simulink model "BLDCmotorControl_FOC_R2017b_fixdt_speedDeriv"  (R2025a)
settings: Solver=FixedStepDiscrete  StartTime=0  StopTime=0.5  FixedStep=Ts  MaxStep=1e-6  RelTol=1e-6  AbsTol=1e-6  EnableMultiTasking=on
PreLoadFcn:
  | addpath(genpath('01_Libraries'));
  | addpath(genpath('02_Figures'));
InitFcn:
  | init_model;
undefined symbols (not defined in the file): a_elecAngle, b_DCLinkCurrAvail, b_fieldWeakEna, b_selPhaABCurrMeas, cf_currFilt, cf_speedCoef, CTRL_COM, DiscIntNeverNeededParam, dV_openRate, DWORK0, DWORK1, DWORK2, DWORK3, dz_cntTrnsDetHi, dz_cntTrnsDetLo, i_max, i_qMax_M1, i_thresOutlier, id_fieldWeak_M1, id_Kb, id_Ki, id_Kp, iq_Kb, iq_Ki, iq_Kp, iq_KpLimProt, n_commAcvLo, n_commDeacvHi, n_Kb, n_Ki, n_Kp, n_KpLimProt, n_max, n_stdStillDet, OPEN_MODE, r_cos_M1, r_sin_M1, r_whl, SPD_MODE, TRQ_MODE, Ts, Ts_ctrl, V_dMax, V_max, V_min, V_qMax_M1, vec_hallToPos, VLT_MODE, z_commutMap_M1, z_ctrlModReq, z_ctrlTypSel, z_maxCntRst
libraries: simulink x11, BLDC_controller_Lib x9, spsVoltageMeasurementLib x2, simulink_extras x1, spsControlledVoltageSourceLib x1, spsPermanentMagnetSynchronousMachineLib x1, spsUniversalBridgeLib x1, spspowerguiLib x1, eePwmGenerator x1, SignalEditorBlockLib x1
(part 3 of 3)

== system BLDCmotorControl_FOC_R2017b_fixdt_speedDeriv/BLDC_controller/BLDC_controller/F03_Field_Oriented_Control/Open_Mode ==
  note: This will reduce the control command to 0 with a predefined rate.
  V_qPrev : Inport
  Action Port : ActionPort  InitializeStates=reset  ActionPortLabel=default: { }
  Constant23 : Constant  Value=0  OutDataTypeStr=Inherit: Inherit via back propagation
  Data Type Conversion : DataTypeConversion  OutDataTypeStr=fixdt(1,28,16)  SaturateOnIntegerOverflow=off  RndMeth=Floor
  Gain3 : Gain  Tag=struct('comment',struct('text','','placement',1),'logdata',struct('maxnumvals',inf,'plotchannels',[],'loggingmode',3,'channels',1),'output',struct('variable','','description','','name','$S_$B','width',1,'address','','max',NaN,'min',NaN,'class','default','type','CONTINUOUS','scaling','','lsb',1,'offset',0,'arb',0,'freeze',1,'unit','','autoscalingmode',1,'lowerheadroom',1,'upperheadroom',1,'headroomunit','bit','keepdatatype',1,'checkmin',0,'checkmax',0,'castoutput',0,'show',0),'gain',struct('variable','','description','','name','$S_$B_gain','width',1,'address','','max',NaN,'min',NaN,'class','default','type','CONTINUOUS','scaling','','lsb',1,'offset',0,'arb',0,'freeze',1,'unit','','keepdatatype',1,'value','1','scalar',0,'tolerance',1),'scalingvalid',0,'date',730486)  Gain=-1  RndMeth=Zero  OutDataTypeStr=Inherit: Same as input
  Rate_Limiter : BLDC_controller_Lib/Rate_Limiter  SystemSampleTime=-1  VariantActivationTime=update diagram  EmptyChoice=off  PassThrough=off  PassThroughVariantControl=(default)  EmptyChoiceVariantControl=(default)  AllowFlexibleInterface=on  Latency=0  AutoFrameSizeCalculation=off
  dV_openRate : Constant  Value=dV_openRate  OutDataTypeStr=fixdt(1,28,16)
  for merge : Gain  Tag=struct('comment',struct('text','','placement',1),'logdata',struct('maxnumvals',inf,'plotchannels',[],'loggingmode',3,'channels',1),'output',struct('variable','','description','','name','$S_$B','width',1,'address','','max',NaN,'min',NaN,'class','default','type','CONTINUOUS','scaling','','lsb',1,'offset',0,'arb',0,'freeze',1,'unit','','autoscalingmode',1,'lowerheadroom',1,'upperheadroom',1,'headroomunit','bit','keepdatatype',1,'checkmin',0,'checkmax',0,'castoutput',0,'show',0),'gain',struct('variable','','description','','name','$S_$B_gain','width',1,'address','','max',NaN,'min',NaN,'class','default','type','CONTINUOUS','scaling','','lsb',1,'offset',0,'arb',0,'freeze',1,'unit','','keepdatatype',1,'value','1','scalar',0,'tolerance',1),'scalingvalid',0,'date',730486)  OutDataTypeStr=fixdt(1,16,4)  RndMeth=Zero
  rising_edge_init : BLDC_controller_Lib/rising_edge_init
  V_qOpen : Outport  VectorParamsAs1DForOutWhenUnconnected=off
  wires:
  V_qPrev/1 -> [V_qPrev]
  Constant23/1 -> Rate_Limiter/1
  rising_edge_init/1 -> Rate_Limiter/3
  Gain3/1 -> Rate_Limiter/5
  dV_openRate/1 -> Gain3/1, Rate_Limiter/4
  for merge/1 -> [V_qOpen]
  [V_qOpen] -> V_qOpen/1
  Rate_Limiter/1 -> for merge/1
  [V_qPrev] -> Data Type Conversion/1
  Data Type Conversion/1 -> Rate_Limiter/2

== system BLDCmotorControl_FOC_R2017b_fixdt_speedDeriv/BLDC_controller/BLDC_controller/F03_Field_Oriented_Control/Outliers_Removal_and_Filtering ==
  i_qRaw : Inport
  i_dRaw : Inport  Port=2
  i_DCLink : Inport  Port=3
  DCLink_Current_Available : Subsystem
  DCLink_Current_NOT_Available : Subsystem
  If1 : If  IfExpression=u1 ~= 0
  Merge : Merge
  Merge1 : Merge
  b_DCLinkCurrAvail : Constant  Value=b_DCLinkCurrAvail  OutDataTypeStr=boolean
  i_q : Outport  VectorParamsAs1DForOutWhenUnconnected=off
  i_d : Outport  Port=2  VectorParamsAs1DForOutWhenUnconnected=off
  wires:
  [i_d] -> i_d/1
  [i_q] -> i_q/1
  i_qRaw/1 -> [i_qRaw]
  i_dRaw/1 -> [i_dRaw]
  [i_qRaw] -> DCLink_Current_NOT_Available/1(i_qRaw)
  [i_dRaw] -> DCLink_Current_NOT_Available/2(i_dRaw)
  If1/1 -> DCLink_Current_Available/Action
  i_DCLink/1 -> [i_DCLink]
  [i_dRaw] -> DCLink_Current_Available/2(i_dRaw)
  [i_qRaw] -> DCLink_Current_Available/1(i_qRaw)
  [i_DCLink] -> DCLink_Current_Available/3(i_DCLink)
  b_DCLinkCurrAvail/1 -> If1/1
  DCLink_Current_NOT_Available/1(i_qNoDCLink) -> [i_qNoDCLink]
  DCLink_Current_NOT_Available/2(i_dNoDCLink) -> [i_dNoDCLink]
  DCLink_Current_Available/1(i_qDCLink) -> [i_qDCLink]
  DCLink_Current_Available/2(i_dDCLink) -> [i_dDCLink]
  Merge1/1 -> [i_d]
  If1/2 -> DCLink_Current_NOT_Available/Action
  [i_qNoDCLink] -> Merge/2
  [i_qDCLink] -> Merge/1
  [i_dDCLink] -> Merge1/1
  [i_dNoDCLink] -> Merge1/2
  Merge/1 -> [i_q]

== system BLDCmotorControl_FOC_R2017b_fixdt_speedDeriv/BLDC_controller/BLDC_controller/F03_Field_Oriented_Control/Park_Transform ==
  note: Park Transform:
      | i_q = -i_alpha*sin(angle) + i_beta*cos(angle)
      | i_d = i_alpha*cos(angle) + i_beta*sin(angle)
  i_apha : Inport
  i_beta : Inport  Port=2
  r_sin : Inport  Port=3
  r_cos : Inport  Port=4
  Divide{1..4} (4 alike) : Product  Inputs=**  RndMeth=Simplest
  Sum1 : Sum  OutDataTypeStr=fixdt(1,16,4)  RndMeth=Simplest  SaturateOnIntegerOverflow=on
  Sum6 : Sum  Inputs=-+  OutDataTypeStr=fixdt(1,16,4)  RndMeth=Simplest  SaturateOnIntegerOverflow=on
  i_q : Outport  VectorParamsAs1DForOutWhenUnconnected=off
  i_d : Outport  Port=2  VectorParamsAs1DForOutWhenUnconnected=off
  wires:
  r_sin/1 -> [r_sin]
  i_beta/1 -> [i_beta]
  i_apha/1 -> [i_apha]
  r_cos/1 -> [r_cos]
  [r_sin] -> Divide4/2
  [i_apha] -> Divide4/1
  Divide4/1 -> Sum6/1
  Divide1/1 -> Sum6/2
  [i_beta] -> Divide1/1
  [r_cos] -> Divide1/2
  Sum6/1 -> i_q/1
  Divide2/1 -> Sum1/1
  [i_apha] -> Divide2/1
  [r_cos] -> Divide2/2
  Divide3/1 -> Sum1/2
  [i_beta] -> Divide3/1
  [r_sin] -> Divide3/2
  Sum1/1 -> i_d/1

== system BLDCmotorControl_FOC_R2017b_fixdt_speedDeriv/BLDC_controller/BLDC_controller/F03_Field_Oriented_Control/Preliminary_Calculations ==
  note: Sine/Cosine Look-up Tables
  note: Field Weakening map as a function of the Motor Speed
  note: FOC Field weakening
  note: Note: The Sine and Cosine maps are shifted in phase by 30 deg to align with the Hall sensors position.
  a_elecAngle : Inport
  n_motAbs : Inport  Port=2
  Data Type Conversion : DataTypeConversion  OutDataTypeStr=fixdt(1,16,4)  SaturateOnIntegerOverflow=off  RndMeth=Floor
  Switch_PhaAdv1 : Switch  Criteria=u2 ~= 0  OutDataTypeStr=Inherit: Inherit via back propagation  RndMeth=Zero  SaturateOnIntegerOverflow=off  InputSameDT=off
  a_elecAngle_XA : PreLookup  BreakpointsData=a_elecAngle_XA  IndexSearchMethod=Evenly spaced points  BeginIndexSearchUsingPreviousIndexResult=on  IndexDataTypeStr=uint8  FractionDataTypeStr=fixdt(0,16,14)  RndMeth=Simplest
  a_elecPeriod2 : Constant  Value=0  OutDataTypeStr=Inherit: Inherit via back propagation
  b_fieldWeakEna : Constant  Value=b_fieldWeakEna  OutDataTypeStr=boolean
  id_fieldWeak_M1 : Interpolation_n-D  NumberOfTableDimensions=1  Table=id_fieldWeak_M1  ExtrapMethod=Clip  OutDataTypeStr=fixdt(0,10,0)  InternalRulePriority=Speed  RndMeth=Simplest
      settings: InputPortMap=u0,u1
  n_fieldWeak_XA : PreLookup  BreakpointsData=n_fieldWeak_XA  IndexSearchMethod=Evenly spaced points  BeginIndexSearchUsingPreviousIndexResult=on  IndexDataTypeStr=uint8  FractionDataTypeStr=fixdt(0,16,14)  RndMeth=Simplest
  r_cos_M1 : Interpolation_n-D  NumberOfTableDimensions=1  Table=r_cos_M1  ExtrapMethod=Clip  OutDataTypeStr=fixdt(1,16,14)  InternalRulePriority=Speed  RndMeth=Simplest
      settings: InputPortMap=u0,u1
  r_sin_M1 : Interpolation_n-D  NumberOfTableDimensions=1  Table=r_sin_M1  ExtrapMethod=Clip  OutDataTypeStr=fixdt(1,16,14)  InternalRulePriority=Speed  RndMeth=Simplest
      settings: InputPortMap=u0,u1
  r_sin : Outport  VectorParamsAs1DForOutWhenUnconnected=off
  r_cos : Outport  Port=2  VectorParamsAs1DForOutWhenUnconnected=off
  i_dTgt : Outport  Port=3  VectorParamsAs1DForOutWhenUnconnected=off
  wires:
  a_elecAngle_XA/2 -> r_sin_M1/2, r_cos_M1/2
  a_elecAngle_XA/1 -> r_cos_M1/1, r_sin_M1/1
  r_sin_M1/1 -> r_sin/1
  a_elecAngle/1 -> a_elecAngle_XA/1
  r_cos_M1/1 -> r_cos/1
  n_fieldWeak_XA/1 -> id_fieldWeak_M1/1
  n_fieldWeak_XA/2 -> id_fieldWeak_M1/2
  id_fieldWeak_M1/1 -> Data Type Conversion/1
  n_motAbs/1 -> n_fieldWeak_XA/1
  b_fieldWeakEna/1 -> Switch_PhaAdv1/2
  a_elecPeriod2/1 -> Switch_PhaAdv1/3
  Switch_PhaAdv1/1 -> i_dTgt/1
  Data Type Conversion/1 -> Switch_PhaAdv1/1

== system BLDCmotorControl_FOC_R2017b_fixdt_speedDeriv/BLDC_controller/BLDC_controller/F03_Field_Oriented_Control/Speed_Mode ==
  r_DC : Inport
  V_qMax : Inport  Port=2
  V_qMin : Inport  Port=3
  n_mot : Inport  Port=4
  n_max : Inport  Port=5
  n_min : Inport  Port=6
  i_qLimProt : Inport  Port=7
  Action Port : ActionPort  InitializeStates=reset  ActionPortLabel=case: { }
  Gain5 : Gain  Tag=struct('comment',struct('text','','placement',1),'logdata',struct('maxnumvals',inf,'plotchannels',[],'loggingmode',3,'channels',1),'output',struct('variable','','description','','name','$S_$B','width',1,'address','','max',NaN,'min',NaN,'class','default','type','CONTINUOUS','scaling','','lsb',1,'offset',0,'arb',0,'freeze',1,'unit','','autoscalingmode',1,'lowerheadroom',1,'upperheadroom',1,'headroomunit','bit','keepdatatype',1,'checkmin',0,'checkmax',0,'castoutput',0,'show',0),'gain',struct('variable','','description','','name','$S_$B_gain','width',1,'address','','max',NaN,'min',NaN,'class','default','type','CONTINUOUS','scaling','','lsb',1,'offset',0,'arb',0,'freeze',1,'unit','','keepdatatype',1,'value','1','scalar',0,'tolerance',1),'scalingvalid',0,'date',730486)  Gain=-1  OutDataTypeStr=fixdt(1,16,4)  RndMeth=Zero  ParamDataTypeStr=Inherit: Same as input
  PI_backCalc_fixdt_n : BLDC_controller_Lib/PI_backCalc_fixdt  SystemSampleTime=-1  VariantActivationTime=update diagram  EmptyChoice=off  PassThrough=off  PassThroughVariantControl=(default)  EmptyChoiceVariantControl=(default)  AllowFlexibleInterface=on  Latency=0  AutoFrameSizeCalculation=off
  Saturation Dynamic1 : simulink/Discontinuities/Saturation Dynamic  OutMin=[]  OutMax=[]  OutDataTypeStr=Inherit: Same as second input  OutDataType=fixdt(1, 16)  OutScaling=2^-10  DoSatur=off
  Sum1 : Sum  RndMeth=Simplest
  Sum3 : Sum  Inputs=|+-  RndMeth=Simplest
  a_elecPeriod11 : Constant  Value=n_Kb  OutDataTypeStr=fixdt(0,16,16)
  a_elecPeriod15 : Constant  Value=n_Kp  OutDataTypeStr=fixdt(0,16,8)
  a_elecPeriod20 : Constant  Value=n_Ki  VectorParams1D=off  OutDataTypeStr=fixdt(0,16,16)
  V_qSpd : Outport  VectorParamsAs1DForOutWhenUnconnected=off
  wires:
  [V_qMin] -> PI_backCalc_fixdt_n/6
  [V_qMax] -> PI_backCalc_fixdt_n/5
  a_elecPeriod20/1 -> PI_backCalc_fixdt_n/3
  a_elecPeriod11/1 -> PI_backCalc_fixdt_n/4
  a_elecPeriod15/1 -> PI_backCalc_fixdt_n/2
  [n_mot] -> Sum3/2
  Sum3/1 -> PI_backCalc_fixdt_n/1
  r_DC/1 -> [r_DC]
  V_qMax/1 -> [V_qMax]
  V_qMin/1 -> [V_qMin]
  n_mot/1 -> [n_mot]
  PI_backCalc_fixdt_n/1 -> Sum1/1
  [V_qSpd] -> V_qSpd/1
  Gain5/1 -> [V_qSpd]
  [n_min] -> Saturation Dynamic1/3
  [n_max] -> Saturation Dynamic1/1
  [r_DC] -> Saturation Dynamic1/2
  Saturation Dynamic1/1 -> Sum3/1
  n_min/1 -> [n_min]
  n_max/1 -> [n_max]
  Sum1/1 -> Gain5/1
  i_qLimProt/1 -> [i_qLimProt]
  [i_qLimProt] -> Sum1/2

== system BLDCmotorControl_FOC_R2017b_fixdt_speedDeriv/BLDC_controller/BLDC_controller/F03_Field_Oriented_Control/Torque_Mode ==
  r_DC : Inport
  V_qMax : Inport  Port=2
  V_qMin : Inport  Port=3
  i_q : Inport  Port=4
  i_qMax : Inport  Port=5
  i_qMin : Inport  Port=6
  n_limProt : Inport  Port=7
  Action Port : ActionPort  InitializeStates=reset  ActionPortLabel=case: { }
  PI_backCalc_fixdt_Iq : BLDC_controller_Lib/PI_backCalc_fixdt  SystemSampleTime=-1  VariantActivationTime=update diagram  EmptyChoice=off  PassThrough=off  PassThroughVariantControl=(default)  EmptyChoiceVariantControl=(default)  AllowFlexibleInterface=on  Latency=0  AutoFrameSizeCalculation=off
  Saturation Dynamic : simulink/Discontinuities/Saturation Dynamic  OutMin=[]  OutMax=[]  OutDataTypeStr=Inherit: Same as second input  OutDataType=fixdt(1, 16)  OutScaling=2^-10  DoSatur=off
  Sum1 : Sum  Inputs=|+-  RndMeth=Simplest
  Sum2 : Sum  RndMeth=Simplest
  a_elecPeriod10 : Constant  Value=iq_Kb  OutDataTypeStr=fixdt(0,16,16)
  a_elecPeriod12 : Constant  Value=iq_Kp  OutDataTypeStr=fixdt(0,16,8)
  a_elecPeriod13 : Constant  Value=iq_Ki  OutDataTypeStr=fixdt(0,16,16)
  due_to_conv : Gain  Tag=struct('comment',struct('text','','placement',1),'logdata',struct('maxnumvals',inf,'plotchannels',[],'loggingmode',3,'channels',1),'output',struct('variable','','description','','name','$S_$B','width',1,'address','','max',NaN,'min',NaN,'class','default','type','CONTINUOUS','scaling','','lsb',1,'offset',0,'arb',0,'freeze',1,'unit','','autoscalingmode',1,'lowerheadroom',1,'upperheadroom',1,'headroomunit','bit','keepdatatype',1,'checkmin',0,'checkmax',0,'castoutput',0,'show',0),'gain',struct('variable','','description','','name','$S_$B_gain','width',1,'address','','max',NaN,'min',NaN,'class','default','type','CONTINUOUS','scaling','','lsb',1,'offset',0,'arb',0,'freeze',1,'unit','','keepdatatype',1,'value','1','scalar',0,'tolerance',1),'scalingvalid',0,'date',730486)  Gain=-1  OutDataTypeStr=fixdt(1,16,3)  RndMeth=Zero  ParamDataTypeStr=Inherit: Same as input
  for merge : Gain  Tag=struct('comment',struct('text','','placement',1),'logdata',struct('maxnumvals',inf,'plotchannels',[],'loggingmode',3,'channels',1),'output',struct('variable','','description','','name','$S_$B','width',1,'address','','max',NaN,'min',NaN,'class','default','type','CONTINUOUS','scaling','','lsb',1,'offset',0,'arb',0,'freeze',1,'unit','','autoscalingmode',1,'lowerheadroom',1,'upperheadroom',1,'headroomunit','bit','keepdatatype',1,'checkmin',0,'checkmax',0,'castoutput',0,'show',0),'gain',struct('variable','','description','','name','$S_$B_gain','width',1,'address','','max',NaN,'min',NaN,'class','default','type','CONTINUOUS','scaling','','lsb',1,'offset',0,'arb',0,'freeze',1,'unit','','keepdatatype',1,'value','1','scalar',0,'tolerance',1),'scalingvalid',0,'date',730486)  RndMeth=Zero  OutDataTypeStr=Inherit: Same as input  ParamDataTypeStr=Inherit: Same as input
  V_qTrq : Outport  VectorParamsAs1DForOutWhenUnconnected=off
  wires:
  a_elecPeriod13/1 -> PI_backCalc_fixdt_Iq/3
  [r_DC] -> Sum2/1
  Saturation Dynamic/1 -> Sum1/1
  [V_qMax] -> PI_backCalc_fixdt_Iq/5
  [V_qMin] -> PI_backCalc_fixdt_Iq/6
  [i_q] -> Sum1/2
  Sum1/1 -> PI_backCalc_fixdt_Iq/1
  a_elecPeriod10/1 -> PI_backCalc_fixdt_Iq/4
  a_elecPeriod12/1 -> PI_backCalc_fixdt_Iq/2
  V_qMax/1 -> [V_qMax]
  r_DC/1 -> [r_DC]
  V_qMin/1 -> [V_qMin]
  i_q/1 -> [i_q]
  [V_qTrq] -> V_qTrq/1
  PI_backCalc_fixdt_Iq/1 -> for merge/1
  for merge/1 -> [V_qTrq]
  i_qMin/1 -> [i_qMin]
  i_qMax/1 -> [i_qMax]
  [i_qMin] -> Saturation Dynamic/3
  [i_qMax] -> Saturation Dynamic/1
  due_to_conv/1 -> Saturation Dynamic/2
  [n_limProt] -> Sum2/2
  n_limProt/1 -> [n_limProt]
  Sum2/1 -> due_to_conv/1

== system BLDCmotorControl_FOC_R2017b_fixdt_speedDeriv/BLDC_controller/BLDC_controller/F03_Field_Oriented_Control/Vd_Calculation ==
  i_dTgt : Inport
  i_d : Inport  Port=2
  V_dMax : Inport  Port=3
  V_dMin : Inport  Port=4
  i_dMax : Inport  Port=5
  i_dMin : Inport  Port=6
  Action Port : ActionPort  InitializeStates=reset  ActionPortLabel=if { }
  PI_backCalc_fixdt_Id : BLDC_controller_Lib/PI_backCalc_fixdt  SystemSampleTime=-1  VariantActivationTime=update diagram  EmptyChoice=off  PassThrough=off  PassThroughVariantControl=(default)  EmptyChoiceVariantControl=(default)  AllowFlexibleInterface=on  Latency=0  AutoFrameSizeCalculation=off
  Saturation Dynamic : simulink/Discontinuities/Saturation Dynamic  OutMin=[]  OutMax=[]  OutDataTypeStr=Inherit: Same as second input  OutDataType=fixdt(1, 16)  OutScaling=2^-10  DoSatur=off
  Sum3 : Sum  Inputs=|+-  RndMeth=Simplest
  a_elecPeriod11 : Constant  Value=id_Kb  OutDataTypeStr=fixdt(0,16,16)
  a_elecPeriod6 : Constant  Value=id_Kp  OutDataTypeStr=fixdt(0,16,8)
  a_elecPeriod7 : Constant  Value=id_Ki  OutDataTypeStr=fixdt(0,16,16)
  V_d : Outport  OutputWhenDisabled=reset  InitialOutput=0  VectorParamsAs1DForOutWhenUnconnected=off
  wires:
  a_elecPeriod6/1 -> PI_backCalc_fixdt_Id/2
  Sum3/1 -> PI_backCalc_fixdt_Id/1
  [V_dMin] -> PI_backCalc_fixdt_Id/6
  [V_dMax] -> PI_backCalc_fixdt_Id/5
  a_elecPeriod7/1 -> PI_backCalc_fixdt_Id/3
  a_elecPeriod11/1 -> PI_backCalc_fixdt_Id/4
  PI_backCalc_fixdt_Id/1 -> [V_d]
  [i_d] -> Sum3/2
  [i_dTgt] -> Saturation Dynamic/2
  [V_d] -> V_d/1
  i_dTgt/1 -> [i_dTgt]
  i_d/1 -> [i_d]
  V_dMin/1 -> [V_dMin]
  V_dMax/1 -> [V_dMax]
  i_dMax/1 -> [i_dMax]
  i_dMin/1 -> [i_dMin]
  Saturation Dynamic/1 -> Sum3/1
  [i_dMax] -> Saturation Dynamic/1
  [i_dMin] -> Saturation Dynamic/3

== system BLDCmotorControl_FOC_R2017b_fixdt_speedDeriv/BLDC_controller/BLDC_controller/F03_Field_Oriented_Control/Voltage_Mode ==
  r_DC : Inport
  V_qMax : Inport  Port=2
  V_qMin : Inport  Port=3
  i_qLimProt : Inport  Port=4
  n_limProt : Inport  Port=5
  Action Port : ActionPort  InitializeStates=reset  ActionPortLabel=case: { }
  Saturation Dynamic1 : simulink/Discontinuities/Saturation Dynamic  OutMin=[]  OutMax=[]  OutDataTypeStr=Inherit: Same as second input  OutDataType=fixdt(1, 16)  OutScaling=2^-10  DoSatur=off
  Sum3 : Sum  Inputs=+++  RndMeth=Simplest
  due_to_conv : Gain  Tag=struct('comment',struct('text','','placement',1),'logdata',struct('maxnumvals',inf,'plotchannels',[],'loggingmode',3,'channels',1),'output',struct('variable','','description','','name','$S_$B','width',1,'address','','max',NaN,'min',NaN,'class','default','type','CONTINUOUS','scaling','','lsb',1,'offset',0,'arb',0,'freeze',1,'unit','','autoscalingmode',1,'lowerheadroom',1,'upperheadroom',1,'headroomunit','bit','keepdatatype',1,'checkmin',0,'checkmax',0,'castoutput',0,'show',0),'gain',struct('variable','','description','','name','$S_$B_gain','width',1,'address','','max',NaN,'min',NaN,'class','default','type','CONTINUOUS','scaling','','lsb',1,'offset',0,'arb',0,'freeze',1,'unit','','keepdatatype',1,'value','1','scalar',0,'tolerance',1),'scalingvalid',0,'date',730486)  Gain=-1  OutDataTypeStr=fixdt(1,16,4)  RndMeth=Zero  ParamDataTypeStr=Inherit: Same as input
  V_qVlt : Outport  VectorParamsAs1DForOutWhenUnconnected=off
  wires:
  r_DC/1 -> [r_DC]
  [V_qMin] -> Saturation Dynamic1/3
  [V_qMax] -> Saturation Dynamic1/1
  [V_qVlt] -> V_qVlt/1
  V_qMax/1 -> [V_qMax]
  V_qMin/1 -> [V_qMin]
  Saturation Dynamic1/1 -> due_to_conv/1
  i_qLimProt/1 -> [i_qLimProt]
  [i_qLimProt] -> Sum3/2
  n_limProt/1 -> [n_limProt]
  [n_limProt] -> Sum3/3
  Sum3/1 -> Saturation Dynamic1/2
  due_to_conv/1 -> [V_qVlt]
  [r_DC] -> Sum3/1

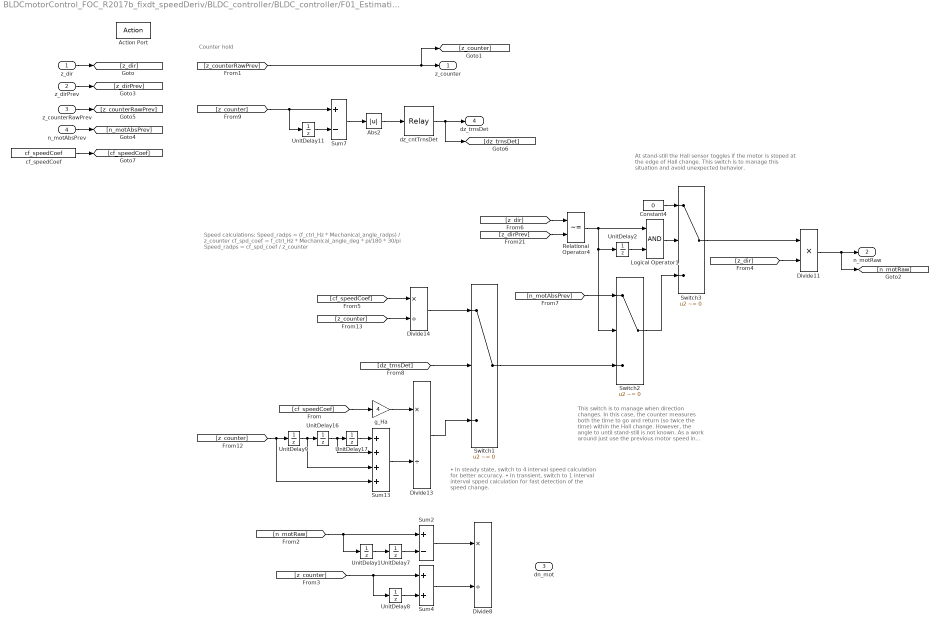
== system BLDCmotorControl_FOC_R2017b_fixdt_speedDeriv/BLDC_controller/BLDC_controller/F01_Estimations/F01_04_Speed_Estimation/Raw_Motor_Speed_Estimation ==
  note: Speed calculations:
      | Speed_radps = (f_ctrl_Hz * Mechanical_angle_radps) / z_counter
      | cf_spd_coef = f_ctrl_Hz * Mechanical_angle_deg * pi/180 * 30/pi
      | Speed_radps = cf_spd_coef / z_counter
  note: Counter hold
  note: • In steady state, switch to 4 interval speed calculation for better accuracy.
      | • In transient, switch to 1 interval interval spped calculation for fast detection of the speed change.
  note: This switch is to manage when direction changes. In this case, the counter measures both the time to go and return (so twice the time) within the Hall change. However, the angle to until stand-still is not known. As a work around just use the previous motor speed in absolute value.
  note: At stand-still the Hall sensor toggles if the motor is stoped at the edge of Hall change. This switch is to manage this situation and avoid unexpected behavior.
  z_dir : Inport
  z_dirPrev : Inport  Port=2
  z_counterRawPrev : Inport  Port=3
  n_motAbsPrev : Inport  Port=4
  Action Port : ActionPort  ActionPortLabel=if(u1 ~= 0)
  Abs2 : Abs  OutDataTypeStr=Inherit: Inherit via back propagation  RndMeth=Zero  SaturateOnIntegerOverflow=off
  Constant4 : Constant  Value=0  OutDataTypeStr=Inherit: Inherit via back propagation
  Divide11 : Product  Inputs=**  RndMeth=Simplest  OutDataTypeStr=Inherit: Same as first input
  Divide13 : Product  Inputs=*/  OutDataTypeStr=fixdt(1,16,4)  RndMeth=Simplest
  Divide14 : Product  Inputs=*/  OutDataTypeStr=fixdt(1,16,4)  RndMeth=Simplest
  Divide8 : Product  Inputs=*/  OutDataTypeStr=fixdt(1,16,6)  RndMeth=Simplest  SaturateOnIntegerOverflow=on
  Logical Operator1 : Logic  AllPortsSameDT=off  OutDataTypeStr=boolean
  Relational Operator4 : RelationalOperator  Operator=~=  OutDataTypeStr=boolean  RndMeth=Simplest  InputSameDT=off
  Sum13 : Sum  Inputs=++++  InputSameDT=on  RndMeth=Simplest  OutDataTypeStr=Inherit: Same as first input
  Sum2 : Sum  Inputs=+-  RndMeth=Simplest  OutDataTypeStr=Inherit: Same as first input
  Sum4 : Sum  RndMeth=Simplest  OutDataTypeStr=Inherit: Same as first input
  Sum7 : Sum  Inputs=+-  InputSameDT=on  RndMeth=Simplest  OutDataTypeStr=Inherit: Same as first input
  Switch1 : Switch  Tag=struct('comment',struct('text','','placement',1),'logdata',struct('maxnumvals',inf,'plotchannels',[],'loggingmode',3,'channels',1),'output',struct('variable','','description','','name','$S_$B','width',1,'address','','max',NaN,'min',NaN,'class','default','type','CONTINUOUS','scaling','','lsb',1,'offset',0,'arb',0,'freeze',1,'unit','','autoscalingmode',1,'lowerheadroom',1,'upperheadroom',1,'headroomunit','bit','keepdatatype',1,'checkmin',0,'checkmax',0,'castoutput',0,'show',0),'threshold',struct('variable','','description','','name','$S_$B_threshold','width',1,'address','','max',NaN,'min',NaN,'class','default','type','CONTINUOUS','scaling','','lsb',1,'offset',0,'arb',0,'freeze',1,'unit','','keepdatatype',1,'value','0','scalar',0,'criteria',3),'scalingvalid',0,'date',733087.49614628474,'inheritscaling',0)  Criteria=u2 ~= 0
      settings: AttributesFormatString=threshold=%<threshold>\nCriteria : %<Criteria>
  Switch2 : Switch  Tag=struct('comment',struct('text','','placement',1),'logdata',struct('maxnumvals',inf,'plotchannels',[],'loggingmode',3,'channels',1),'output',struct('variable','','description','','name','$S_$B','width',1,'address','','max',NaN,'min',NaN,'class','default','type','CONTINUOUS','scaling','','lsb',1,'offset',0,'arb',0,'freeze',1,'unit','','autoscalingmode',1,'lowerheadroom',1,'upperheadroom',1,'headroomunit','bit','keepdatatype',1,'checkmin',0,'checkmax',0,'castoutput',0,'show',0),'threshold',struct('variable','','description','','name','$S_$B_threshold','width',1,'address','','max',NaN,'min',NaN,'class','default','type','CONTINUOUS','scaling','','lsb',1,'offset',0,'arb',0,'freeze',1,'unit','','keepdatatype',1,'value','0','scalar',0,'criteria',3),'scalingvalid',0,'date',733087.49614628474,'inheritscaling',0)  Criteria=u2 ~= 0
      settings: AttributesFormatString=threshold=%<threshold>\nCriteria : %<Criteria>
  Switch3 : Switch  Tag=struct('comment',struct('text','','placement',1),'logdata',struct('maxnumvals',inf,'plotchannels',[],'loggingmode',3,'channels',1),'output',struct('variable','','description','','name','$S_$B','width',1,'address','','max',NaN,'min',NaN,'class','default','type','CONTINUOUS','scaling','','lsb',1,'offset',0,'arb',0,'freeze',1,'unit','','autoscalingmode',1,'lowerheadroom',1,'upperheadroom',1,'headroomunit','bit','keepdatatype',1,'checkmin',0,'checkmax',0,'castoutput',0,'show',0),'threshold',struct('variable','','description','','name','$S_$B_threshold','width',1,'address','','max',NaN,'min',NaN,'class','default','type','CONTINUOUS','scaling','','lsb',1,'offset',0,'arb',0,'freeze',1,'unit','','keepdatatype',1,'value','0','scalar',0,'criteria',3),'scalingvalid',0,'date',733087.49614628474,'inheritscaling',0)  Criteria=u2 ~= 0
      settings: AttributesFormatString=threshold=%<threshold>\nCriteria : %<Criteria>
  UnitDelay{1..2,7..9,11,16..17} (8 alike) : UnitDelay  SampleTime=-1  HasFrameUpgradeWarning=on
  cf_speedCoef : Constant  Value=cf_speedCoef  OutDataTypeStr=fixdt(0,16,0)
  dz_cntTrnsDet : Relay  OnSwitchValue=dz_cntTrnsDetHi  OffSwitchValue=dz_cntTrnsDetLo  OutDataTypeStr=boolean
  g_Ha : Gain  Gain=4  OutDataTypeStr=Inherit: Inherit via back propagation  RndMeth=Zero  ParamDataTypeStr=Inherit: Same as input
  z_counter : Outport  InitialOutput=z_maxCntRst  VectorParamsAs1DForOutWhenUnconnected=off
  n_motRaw : Outport  Port=2  VectorParamsAs1DForOutWhenUnconnected=off
  dn_mot : Outport  Port=3  VectorParamsAs1DForOutWhenUnconnected=off
  dz_trnsDet : Outport  Port=4  VectorParamsAs1DForOutWhenUnconnected=off
  wires:
  z_dir/1 -> [z_dir]
  z_dirPrev/1 -> [z_dirPrev]
  z_counterRawPrev/1 -> [z_counterRawPrev]
  UnitDelay1/1 -> UnitDelay7/1
  Divide11/1 -> [n_motRaw], n_motRaw/1
  Sum2/1 -> Divide8/1
  [z_counter] -> UnitDelay8/1, Sum4/1
  [n_motRaw] -> Sum2/1, UnitDelay1/1
  UnitDelay7/1 -> Sum2/2
  UnitDelay8/1 -> Sum4/2
  Sum4/1 -> Divide8/2
  [z_dir] -> Divide11/2
  UnitDelay16/1 -> Sum13/2, UnitDelay17/1
  UnitDelay9/1 -> Sum13/3, UnitDelay16/1
  [z_counter] -> Sum13/4, UnitDelay9/1
  [cf_speedCoef] -> g_Ha/1
  Sum13/1 -> Divide13/2
  g_Ha/1 -> Divide13/1
  [z_counter] -> Divide14/2
  [cf_speedCoef] -> Divide14/1
  UnitDelay11/1 -> Sum7/2
  [z_counter] -> Sum7/1, UnitDelay11/1
  Sum7/1 -> Abs2/1
  Abs2/1 -> dz_cntTrnsDet/1
  [dz_trnsDet] -> Switch1/2
  cf_speedCoef/1 -> [cf_speedCoef]
  UnitDelay17/1 -> Sum13/1
  [z_dir] -> Relational Operator4/1
  [z_dirPrev] -> Relational Operator4/2
  UnitDelay2/1 -> Logical Operator1/2
  Relational Operator4/1 -> Switch2/2, UnitDelay2/1, Logical Operator1/1
  Logical Operator1/1 -> Switch3/2
  Switch2/1 -> Switch3/3
  Constant4/1 -> Switch3/1
  Switch3/1 -> Divide11/1
  Switch1/1 -> Switch2/3
  n_motAbsPrev/1 -> [n_motAbsPrev]
  [n_motAbsPrev] -> Switch2/1
  [z_counterRawPrev] -> [z_counter], z_counter/1
  dz_cntTrnsDet/1 -> [dz_trnsDet], dz_trnsDet/1
  Divide14/1 -> Switch1/1
  Divide13/1 -> Switch1/3

== system BLDCmotorControl_FOC_R2017b_fixdt_speedDeriv/BLDC_controller/BLDC_controller/F03_Field_Oriented_Control/Clarke_Transform/Clarke_PhasesAB ==
  note: Clarke Transform:
      | i_alpha = i_phaA
      | i_beta = ((1/sqrt(3))*i_phaA + (2/sqrt(3))*i_phaB)
  i_phaA : Inport
  i_phaB : Inport  Port=2
  Action Port : ActionPort  ActionPortLabel=if(u1 ~= 0)
  Gain2 : Gain  Tag=struct('comment',struct('text','','placement',1),'logdata',struct('maxnumvals',inf,'plotchannels',[],'loggingmode',3,'channels',1),'output',struct('variable','','description','','name','$S_$B','width',1,'address','','max',NaN,'min',NaN,'class','default','type','CONTINUOUS','scaling','','lsb',1,'offset',0,'arb',0,'freeze',1,'unit','','autoscalingmode',1,'lowerheadroom',1,'upperheadroom',1,'headroomunit','bit','keepdatatype',1,'checkmin',0,'checkmax',0,'castoutput',0,'show',0),'gain',struct('variable','','description','','name','$S_$B_gain','width',1,'address','','max',NaN,'min',NaN,'class','default','type','CONTINUOUS','scaling','','lsb',1,'offset',0,'arb',0,'freeze',1,'unit','','keepdatatype',1,'value','1','scalar',0,'tolerance',1),'scalingvalid',0,'date',730486)  Gain=2/sqrt(3)  RndMeth=Zero
  Gain4 : Gain  Tag=struct('comment',struct('text','','placement',1),'logdata',struct('maxnumvals',inf,'plotchannels',[],'loggingmode',3,'channels',1),'output',struct('variable','','description','','name','$S_$B','width',1,'address','','max',NaN,'min',NaN,'class','default','type','CONTINUOUS','scaling','','lsb',1,'offset',0,'arb',0,'freeze',1,'unit','','autoscalingmode',1,'lowerheadroom',1,'upperheadroom',1,'headroomunit','bit','keepdatatype',1,'checkmin',0,'checkmax',0,'castoutput',0,'show',0),'gain',struct('variable','','description','','name','$S_$B_gain','width',1,'address','','max',NaN,'min',NaN,'class','default','type','CONTINUOUS','scaling','','lsb',1,'offset',0,'arb',0,'freeze',1,'unit','','keepdatatype',1,'value','1','scalar',0,'tolerance',1),'scalingvalid',0,'date',730486)  Gain=1/sqrt(3)  RndMeth=Zero
  Sum1 : Sum  OutDataTypeStr=fixdt(1,16,4)  RndMeth=Simplest  SaturateOnIntegerOverflow=on
  for merge : Gain  Tag=struct('comment',struct('text','','placement',1),'logdata',struct('maxnumvals',inf,'plotchannels',[],'loggingmode',3,'channels',1),'output',struct('variable','','description','','name','$S_$B','width',1,'address','','max',NaN,'min',NaN,'class','default','type','CONTINUOUS','scaling','','lsb',1,'offset',0,'arb',0,'freeze',1,'unit','','autoscalingmode',1,'lowerheadroom',1,'upperheadroom',1,'headroomunit','bit','keepdatatype',1,'checkmin',0,'checkmax',0,'castoutput',0,'show',0),'gain',struct('variable','','description','','name','$S_$B_gain','width',1,'address','','max',NaN,'min',NaN,'class','default','type','CONTINUOUS','scaling','','lsb',1,'offset',0,'arb',0,'freeze',1,'unit','','keepdatatype',1,'value','1','scalar',0,'tolerance',1),'scalingvalid',0,'date',730486)  RndMeth=Zero  OutDataTypeStr=Inherit: Same as input  ParamDataTypeStr=Inherit: Same as input
  i_alphaAB : Outport  VectorParamsAs1DForOutWhenUnconnected=off
  i_betaAB : Outport  Port=2  VectorParamsAs1DForOutWhenUnconnected=off
  wires:
  i_phaB/1 -> [i_phaB]
  i_phaA/1 -> [i_phaA]
  [i_phaA] -> for merge/1, Gain4/1
  Gain2/1 -> Sum1/2
  [i_phaB] -> Gain2/1
  Gain4/1 -> Sum1/1
  Sum1/1 -> i_betaAB/1
  for merge/1 -> i_alphaAB/1

== system BLDCmotorControl_FOC_R2017b_fixdt_speedDeriv/BLDC_controller/BLDC_controller/F03_Field_Oriented_Control/Clarke_Transform/Clarke_PhasesBC ==
  note: Clarke Transform:
      | i_alpha = - i_phaB - i_phaC
      | i_beta = (1/sqrt(3)) * (i_phaB - i_phaC)
  i_phaB : Inport
  i_phaC : Inport  Port=2
  Action Port : ActionPort  ActionPortLabel=else
  Gain2 : Gain  Tag=struct('comment',struct('text','','placement',1),'logdata',struct('maxnumvals',inf,'plotchannels',[],'loggingmode',3,'channels',1),'output',struct('variable','','description','','name','$S_$B','width',1,'address','','max',NaN,'min',NaN,'class','default','type','CONTINUOUS','scaling','','lsb',1,'offset',0,'arb',0,'freeze',1,'unit','','autoscalingmode',1,'lowerheadroom',1,'upperheadroom',1,'headroomunit','bit','keepdatatype',1,'checkmin',0,'checkmax',0,'castoutput',0,'show',0),'gain',struct('variable','','description','','name','$S_$B_gain','width',1,'address','','max',NaN,'min',NaN,'class','default','type','CONTINUOUS','scaling','','lsb',1,'offset',0,'arb',0,'freeze',1,'unit','','keepdatatype',1,'value','1','scalar',0,'tolerance',1),'scalingvalid',0,'date',730486)  Gain=1/sqrt(3)  OutDataTypeStr=fixdt(1,16,4)  RndMeth=Zero  SaturateOnIntegerOverflow=on
  Sum1 : Sum  Inputs=--  OutDataTypeStr=fixdt(1,16,4)  RndMeth=Simplest  SaturateOnIntegerOverflow=on
  Sum3 : Sum  Inputs=+-  RndMeth=Simplest
  i_alphaBC : Outport  VectorParamsAs1DForOutWhenUnconnected=off
  i_betaBC : Outport  Port=2  VectorParamsAs1DForOutWhenUnconnected=off
  wires:
  [i_phaC] -> Sum1/2
  [i_phaB] -> Sum1/1
  [i_phaC] -> Sum3/2
  Gain2/1 -> i_betaBC/1
  Sum3/1 -> Gain2/1
  [i_phaB] -> Sum3/1
  Sum1/1 -> i_alphaBC/1
  i_phaB/1 -> [i_phaB]
  i_phaC/1 -> [i_phaC]

== system BLDCmotorControl_FOC_R2017b_fixdt_speedDeriv/BLDC_controller/BLDC_controller/F03_Field_Oriented_Control/Motor_Limitations/Current_Limit_Protection ==
  i_q : Inport
  i_qMax : Inport  Port=2
  i_qMin : Inport  Port=3
  Action Port : ActionPort  InitializeStates=reset  ActionPortLabel=if { }
  Divide4 : Product  Inputs=**  RndMeth=Simplest  OutDataTypeStr=Inherit: Same as first input
  Gain2 : Gain  Tag=struct('comment',struct('text','','placement',1),'logdata',struct('maxnumvals',inf,'plotchannels',[],'loggingmode',3,'channels',1),'output',struct('variable','','description','','name','$S_$B','width',1,'address','','max',NaN,'min',NaN,'class','default','type','CONTINUOUS','scaling','','lsb',1,'offset',0,'arb',0,'freeze',1,'unit','','autoscalingmode',1,'lowerheadroom',1,'upperheadroom',1,'headroomunit','bit','keepdatatype',1,'checkmin',0,'checkmax',0,'castoutput',0,'show',0),'gain',struct('variable','','description','','name','$S_$B_gain','width',1,'address','','max',NaN,'min',NaN,'class','default','type','CONTINUOUS','scaling','','lsb',1,'offset',0,'arb',0,'freeze',1,'unit','','keepdatatype',1,'value','1','scalar',0,'tolerance',1),'scalingvalid',0,'date',730486)  Gain=-1  RndMeth=Zero  SaturateOnIntegerOverflow=on  OutDataTypeStr=Inherit: Same as input  ParamDataTypeStr=Inherit: Same as input
  Kp_iqLimProt : Constant  Value=iq_KpLimProt  OutDataTypeStr=fixdt(0,16,6)
  Saturation Dynamic : simulink/Discontinuities/Saturation Dynamic  OutMin=[]  OutMax=[]  OutDataTypeStr=Inherit: Same as second input  OutDataType=fixdt(1, 16)  OutScaling=2^-10  DoSatur=off
  Sum3 : Sum  Inputs=|+-  RndMeth=Simplest
  i_qLimProt : Outport  VectorParamsAs1DForOutWhenUnconnected=off
  wires:
  Sum3/1 -> Divide4/1
  Gain2/1 -> Sum3/2, Saturation Dynamic/2
  Kp_iqLimProt/1 -> Divide4/2
  Saturation Dynamic/1 -> Sum3/1
  i_qMax/1 -> Saturation Dynamic/1
  i_q/1 -> Gain2/1
  i_qMin/1 -> Saturation Dynamic/3
  Divide4/1 -> i_qLimProt/1

== system BLDCmotorControl_FOC_R2017b_fixdt_speedDeriv/BLDC_controller/BLDC_controller/F03_Field_Oriented_Control/Motor_Limitations/Speed_Limit_Protection ==
  n_mot : Inport
  n_max : Inport  Port=2
  n_min : Inport  Port=3
  Action Port : ActionPort  InitializeStates=reset  ActionPortLabel=if { }
  Divide1 : Product  Inputs=**  RndMeth=Simplest  OutDataTypeStr=Inherit: Same as first input
  Kp_nLimProt : Constant  Value=n_KpLimProt  OutDataTypeStr=fixdt(0,16,6)
  Saturation Dynamic1 : simulink/Discontinuities/Saturation Dynamic  OutMin=[]  OutMax=[]  OutDataTypeStr=Inherit: Same as second input  OutDataType=fixdt(1, 16)  OutScaling=2^-10  DoSatur=off
  Sum1 : Sum  Inputs=|+-  RndMeth=Simplest
  n_limProt : Outport  VectorParamsAs1DForOutWhenUnconnected=off
  wires:
  Saturation Dynamic1/1 -> Sum1/1
  n_min/1 -> Saturation Dynamic1/3
  Sum1/1 -> Divide1/1
  n_max/1 -> Saturation Dynamic1/1
  Kp_nLimProt/1 -> Divide1/2
  n_mot/1 -> Sum1/2, Saturation Dynamic1/2
  Divide1/1 -> n_limProt/1

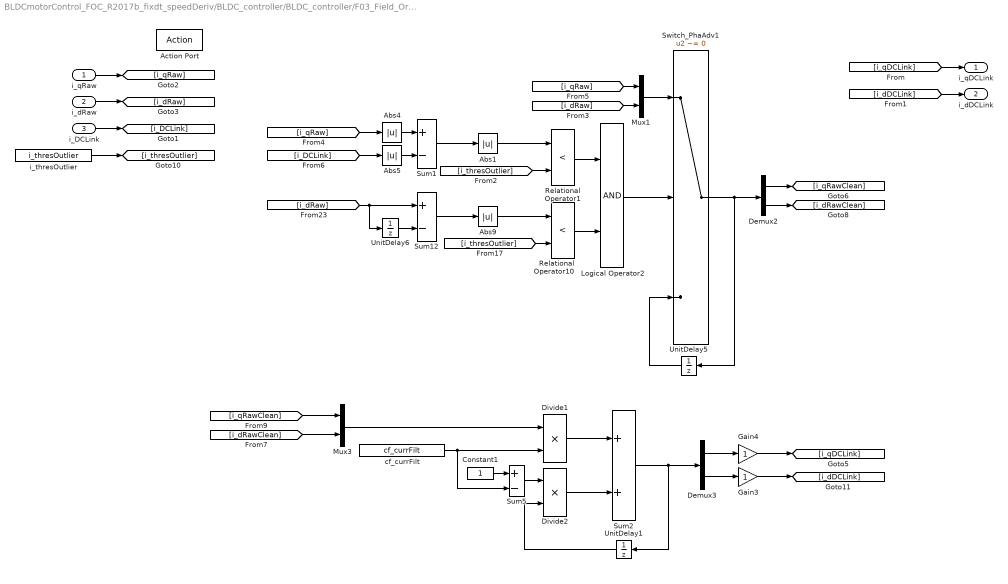
== system BLDCmotorControl_FOC_R2017b_fixdt_speedDeriv/BLDC_controller/BLDC_controller/F03_Field_Oriented_Control/Outliers_Removal_and_Filtering/DCLink_Current_Available ==
  i_qRaw : Inport
  i_dRaw : Inport  Port=2
  i_DCLink : Inport  Port=3
  Action Port : ActionPort  ActionPortLabel=if { }
  Abs{1,4..5,9} (4 alike) : Abs  SaturateOnIntegerOverflow=off
  Constant1 : Constant  OutDataTypeStr=Inherit: Inherit via back propagation
  Demux2 : Demux  Outputs=2
  Demux3 : Demux  Outputs=2
  Divide1 : Product  Inputs=**  RndMeth=Simplest
  Divide2 : Product  Inputs=**  RndMeth=Simplest
  Gain3 : Gain  Tag=struct('comment',struct('text','','placement',1),'logdata',struct('maxnumvals',inf,'plotchannels',[],'loggingmode',3,'channels',1),'output',struct('variable','','description','','name','$S_$B','width',1,'address','','max',NaN,'min',NaN,'class','default','type','CONTINUOUS','scaling','','lsb',1,'offset',0,'arb',0,'freeze',1,'unit','','autoscalingmode',1,'lowerheadroom',1,'upperheadroom',1,'headroomunit','bit','keepdatatype',1,'checkmin',0,'checkmax',0,'castoutput',0,'show',0),'gain',struct('variable','','description','','name','$S_$B_gain','width',1,'address','','max',NaN,'min',NaN,'class','default','type','CONTINUOUS','scaling','','lsb',1,'offset',0,'arb',0,'freeze',1,'unit','','keepdatatype',1,'value','1','scalar',0,'tolerance',1),'scalingvalid',0,'date',730486)  RndMeth=Zero  OutDataTypeStr=Inherit: Same as input  ParamDataTypeStr=Inherit: Same as input
  Gain4 : Gain  Tag=struct('comment',struct('text','','placement',1),'logdata',struct('maxnumvals',inf,'plotchannels',[],'loggingmode',3,'channels',1),'output',struct('variable','','description','','name','$S_$B','width',1,'address','','max',NaN,'min',NaN,'class','default','type','CONTINUOUS','scaling','','lsb',1,'offset',0,'arb',0,'freeze',1,'unit','','autoscalingmode',1,'lowerheadroom',1,'upperheadroom',1,'headroomunit','bit','keepdatatype',1,'checkmin',0,'checkmax',0,'castoutput',0,'show',0),'gain',struct('variable','','description','','name','$S_$B_gain','width',1,'address','','max',NaN,'min',NaN,'class','default','type','CONTINUOUS','scaling','','lsb',1,'offset',0,'arb',0,'freeze',1,'unit','','keepdatatype',1,'value','1','scalar',0,'tolerance',1),'scalingvalid',0,'date',730486)  RndMeth=Zero  OutDataTypeStr=Inherit: Same as input  ParamDataTypeStr=Inherit: Same as input
  Logical Operator2 : Logic  AllPortsSameDT=off  OutDataTypeStr=boolean
  Mux1 : Mux  Inputs=2
  Mux3 : Mux  Inputs=2
  Relational Operator1 : RelationalOperator  Operator=<  OutDataTypeStr=boolean  RndMeth=Simplest  InputSameDT=off
  Relational Operator10 : RelationalOperator  Operator=<  OutDataTypeStr=boolean  RndMeth=Simplest  InputSameDT=off
  Sum1 : Sum  Inputs=+-  RndMeth=Simplest
  Sum12 : Sum  Inputs=+-  RndMeth=Simplest
  Sum2 : Sum  OutDataTypeStr=fixdt(1,16,4)  InputSameDT=on  RndMeth=Simplest
  Sum5 : Sum  Inputs=+-  InputSameDT=on  RndMeth=Simplest  OutDataTypeStr=Inherit: Same as first input
  Switch_PhaAdv1 : Switch  Criteria=u2 ~= 0  OutDataTypeStr=Inherit: Inherit via back propagation  RndMeth=Zero  SaturateOnIntegerOverflow=off  InputSameDT=off
  UnitDelay1 : UnitDelay  SampleTime=-1  HasFrameUpgradeWarning=on
  UnitDelay5 : UnitDelay  SampleTime=-1  HasFrameUpgradeWarning=on
  UnitDelay6 : UnitDelay  SampleTime=-1  HasFrameUpgradeWarning=on
  cf_currFilt : Constant  Value=cf_currFilt  OutDataTypeStr=fixdt(0,16,16)
  i_thresOutlier : Constant  Value=i_thresOutlier  OutDataTypeStr=fixdt(0,16,0)
  i_qDCLink : Outport  VectorParamsAs1DForOutWhenUnconnected=off
  i_dDCLink : Outport  Port=2  VectorParamsAs1DForOutWhenUnconnected=off
  wires:
  Demux2/1 -> [i_qRawClean]
  Demux2/2 -> [i_dRawClean]
  [i_dRaw] -> Mux1/2
  [i_qRaw] -> Mux1/1
  [i_thresOutlier] -> Relational Operator1/2
  Sum1/1 -> Abs1/1
  Abs1/1 -> Relational Operator1/1
  [i_dDCLink] -> i_dDCLink/1
  i_qRaw/1 -> [i_qRaw]
  [i_qDCLink] -> i_qDCLink/1
  i_dRaw/1 -> [i_dRaw]
  i_DCLink/1 -> [i_DCLink]
  Relational Operator1/1 -> Logical Operator2/1
  Mux1/1 -> Switch_PhaAdv1/1
  UnitDelay5/1 -> Switch_PhaAdv1/3
  [i_qRaw] -> Abs4/1
  [i_DCLink] -> Abs5/1
  Switch_PhaAdv1/1 -> Demux2/1, UnitDelay5/1
  Abs5/1 -> Sum1/2
  Abs4/1 -> Sum1/1
  [i_dRaw] -> UnitDelay6/1, Sum12/1
  Abs9/1 -> Relational Operator10/1
  Sum12/1 -> Abs9/1
  [i_thresOutlier] -> Relational Operator10/2
  i_thresOutlier/1 -> [i_thresOutlier]
  Relational Operator10/1 -> Logical Operator2/2
  Gain4/1 -> [i_qDCLink]
  Gain3/1 -> [i_dDCLink]
  Logical Operator2/1 -> Switch_PhaAdv1/2
  UnitDelay6/1 -> Sum12/2
  UnitDelay1/1 -> Divide2/2
  [i_qRawClean] -> Mux3/1
  Divide2/1 -> Sum2/2
  cf_currFilt/1 -> Divide1/2, Sum5/2
  Sum5/1 -> Divide2/1
  [i_dRawClean] -> Mux3/2
  Demux3/2 -> Gain3/1
  Divide1/1 -> Sum2/1
  Demux3/1 -> Gain4/1
  Sum2/1 -> UnitDelay1/1, Demux3/1
  Mux3/1 -> Divide1/1
  Constant1/1 -> Sum5/1

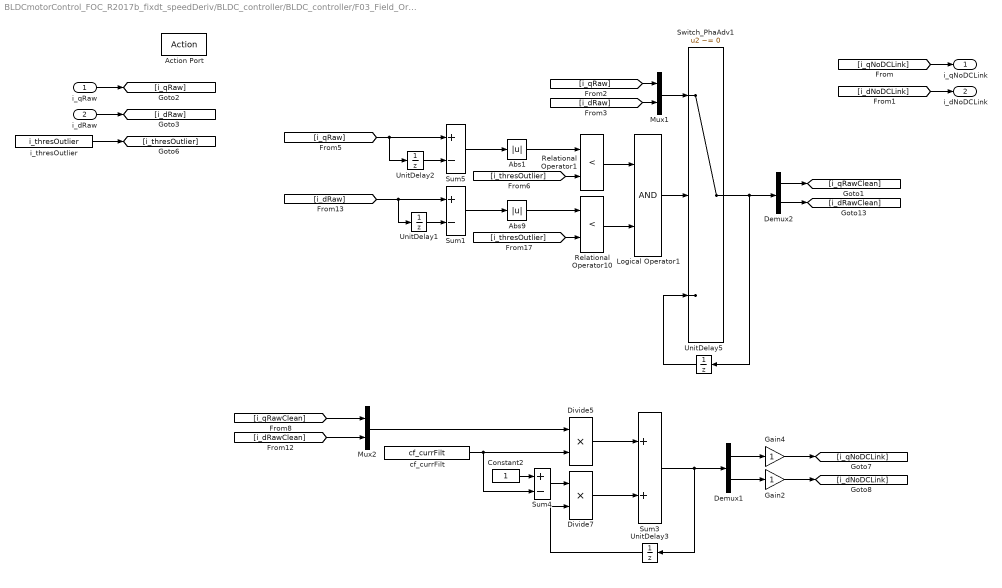
== system BLDCmotorControl_FOC_R2017b_fixdt_speedDeriv/BLDC_controller/BLDC_controller/F03_Field_Oriented_Control/Outliers_Removal_and_Filtering/DCLink_Current_NOT_Available ==
  i_qRaw : Inport
  i_dRaw : Inport  Port=2
  Action Port : ActionPort  ActionPortLabel=else { }
  Abs1 : Abs  SaturateOnIntegerOverflow=off
  Abs9 : Abs  SaturateOnIntegerOverflow=off
  Constant2 : Constant  OutDataTypeStr=Inherit: Inherit via back propagation
  Demux1 : Demux  Outputs=2
  Demux2 : Demux  Outputs=2
  Divide5 : Product  Inputs=**  RndMeth=Simplest
  Divide7 : Product  Inputs=**  RndMeth=Simplest
  Gain2 : Gain  Tag=struct('comment',struct('text','','placement',1),'logdata',struct('maxnumvals',inf,'plotchannels',[],'loggingmode',3,'channels',1),'output',struct('variable','','description','','name','$S_$B','width',1,'address','','max',NaN,'min',NaN,'class','default','type','CONTINUOUS','scaling','','lsb',1,'offset',0,'arb',0,'freeze',1,'unit','','autoscalingmode',1,'lowerheadroom',1,'upperheadroom',1,'headroomunit','bit','keepdatatype',1,'checkmin',0,'checkmax',0,'castoutput',0,'show',0),'gain',struct('variable','','description','','name','$S_$B_gain','width',1,'address','','max',NaN,'min',NaN,'class','default','type','CONTINUOUS','scaling','','lsb',1,'offset',0,'arb',0,'freeze',1,'unit','','keepdatatype',1,'value','1','scalar',0,'tolerance',1),'scalingvalid',0,'date',730486)  RndMeth=Zero  OutDataTypeStr=Inherit: Same as input  ParamDataTypeStr=Inherit: Same as input
  Gain4 : Gain  Tag=struct('comment',struct('text','','placement',1),'logdata',struct('maxnumvals',inf,'plotchannels',[],'loggingmode',3,'channels',1),'output',struct('variable','','description','','name','$S_$B','width',1,'address','','max',NaN,'min',NaN,'class','default','type','CONTINUOUS','scaling','','lsb',1,'offset',0,'arb',0,'freeze',1,'unit','','autoscalingmode',1,'lowerheadroom',1,'upperheadroom',1,'headroomunit','bit','keepdatatype',1,'checkmin',0,'checkmax',0,'castoutput',0,'show',0),'gain',struct('variable','','description','','name','$S_$B_gain','width',1,'address','','max',NaN,'min',NaN,'class','default','type','CONTINUOUS','scaling','','lsb',1,'offset',0,'arb',0,'freeze',1,'unit','','keepdatatype',1,'value','1','scalar',0,'tolerance',1),'scalingvalid',0,'date',730486)  RndMeth=Zero  OutDataTypeStr=Inherit: Same as input  ParamDataTypeStr=Inherit: Same as input
  Logical Operator1 : Logic  AllPortsSameDT=off  OutDataTypeStr=boolean
  Mux1 : Mux  Inputs=2
  Mux2 : Mux  Inputs=2
  Relational Operator1 : RelationalOperator  Operator=<  OutDataTypeStr=boolean  RndMeth=Simplest  InputSameDT=off
  Relational Operator10 : RelationalOperator  Operator=<  OutDataTypeStr=boolean  RndMeth=Simplest  InputSameDT=off
  Sum1 : Sum  Inputs=+-  RndMeth=Simplest
  Sum3 : Sum  OutDataTypeStr=fixdt(1,16,4)  InputSameDT=on  RndMeth=Simplest
  Sum4 : Sum  Inputs=+-  InputSameDT=on  RndMeth=Simplest  OutDataTypeStr=Inherit: Same as first input
  Sum5 : Sum  Inputs=+-  RndMeth=Simplest
  Switch_PhaAdv1 : Switch  Criteria=u2 ~= 0  OutDataTypeStr=Inherit: Inherit via back propagation  RndMeth=Zero  SaturateOnIntegerOverflow=off  InputSameDT=off
  UnitDelay{1..3,5} (4 alike) : UnitDelay  SampleTime=-1  HasFrameUpgradeWarning=on
  cf_currFilt : Constant  Value=cf_currFilt  OutDataTypeStr=fixdt(0,16,16)
  i_thresOutlier : Constant  Value=i_thresOutlier  OutDataTypeStr=fixdt(0,16,0)
  i_qNoDCLink : Outport  VectorParamsAs1DForOutWhenUnconnected=off
  i_dNoDCLink : Outport  Port=2  VectorParamsAs1DForOutWhenUnconnected=off
  wires:
  i_qRaw/1 -> [i_qRaw]
  i_dRaw/1 -> [i_dRaw]
  [i_qNoDCLink] -> i_qNoDCLink/1
  [i_dNoDCLink] -> i_dNoDCLink/1
  Sum5/1 -> Abs1/1
  UnitDelay2/1 -> Sum5/2
  [i_thresOutlier] -> Relational Operator1/2
  Abs1/1 -> Relational Operator1/1
  i_thresOutlier/1 -> [i_thresOutlier]
  Relational Operator1/1 -> Logical Operator1/1
  [i_qRaw] -> Sum5/1, UnitDelay2/1
  Sum1/1 -> Abs9/1
  [i_thresOutlier] -> Relational Operator10/2
  Abs9/1 -> Relational Operator10/1
  Mux1/1 -> Switch_PhaAdv1/1
  [i_dRaw] -> Mux1/2
  Logical Operator1/1 -> Switch_PhaAdv1/2
  UnitDelay5/1 -> Switch_PhaAdv1/3
  [i_qRaw] -> Mux1/1
  Demux2/1 -> [i_qRawClean]
  Switch_PhaAdv1/1 -> Demux2/1, UnitDelay5/1
  Demux2/2 -> [i_dRawClean]
  [i_dRaw] -> UnitDelay1/1, Sum1/1
  UnitDelay1/1 -> Sum1/2
  Relational Operator10/1 -> Logical Operator1/2
  Mux2/1 -> Divide5/1
  Constant2/1 -> Sum4/1
  Demux1/2 -> Gain2/1
  [i_dRawClean] -> Mux2/2
  Demux1/1 -> Gain4/1
  Divide5/1 -> Sum3/1
  Divide7/1 -> Sum3/2
  cf_currFilt/1 -> Divide5/2, Sum4/2
  Sum3/1 -> UnitDelay3/1, Demux1/1
  Sum4/1 -> Divide7/1
  [i_qRawClean] -> Mux2/1
  UnitDelay3/1 -> Divide7/2
  Gain2/1 -> [i_dNoDCLink]
  Gain4/1 -> [i_qNoDCLink]

== stateflow chart BLDCmotorControl_FOC_R2017b_fixdt_speedDeriv/BLDC_controller/BLDC_controller/F02_Control_Mode_Manager/F02_01_Control_Mode_Manager ==
  state OPEN
    entry:
    z_ctrlMod = OPEN_MODE;
  state ACTIVE
    state TORQUE_MODE
      entry:
      z_ctrlMod = TRQ_MODE;
    state SPEED_MODE
      entry:
      z_ctrlMod = SPD_MODE;
    state VOLTAGE_MODE
      entry:
      z_ctrlMod = VLT_MODE;
    (default) -> (junction 7)
    (junction 7) -> TORQUE_MODE [order 1] : [b_toTrqMod]
    (junction 7) -> (junction 8) [order 2]
    (junction 8) -> SPEED_MODE [order 1] : [b_toSpdMod]
    (junction 8) -> (junction 29) [order 2]
    (junction 29) -> VOLTAGE_MODE
  (default) -> OPEN
  OPEN -> ACTIVE : [b_toActive]
  ACTIVE -> OPEN : [b_toOpen]
  data: b_toOpen input boolean; b_toActive input boolean; b_toSpdMod input boolean; z_ctrlMod output uint8; OPEN_MODE constant uint8 =OPEN_MODE; TRQ_MODE constant uint8 =TRQ_MODE; SPD_MODE constant uint8 =SPD_MODE; VLT_MODE constant uint8 =VLT_MODE; b_toTrqMod input boolean
